simulink model "demonstrator"  (Simulink 7.4)
settings: Solver=FixedStepDiscrete  StartTime=0.0  StopTime=10.0  FixedStep=0.001  RelTol=1e-3
libraries: BusImpl x3, AtomicLibrary x1, robot x1, robot2 x1
settings Model: Creator=andrey  LastModifiedBy=andrey
settings SolverCC: AutoInsertRateTranBlk=on
settings DebuggingCC: MultiTaskDSMMsg=warning  MultiTaskCondExecSysMsg=none
settings RTWCC: IncludeERTFirstTime=on

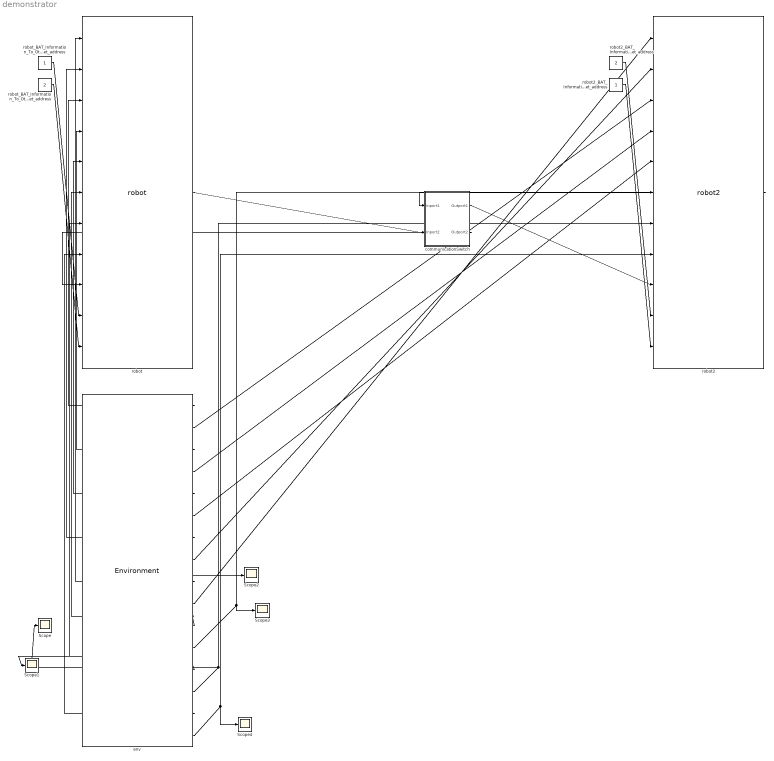
== system demonstrator ==
  Scope{,1..4} (5 alike) : Scope
      Scope settings: YMin=-1  YMax=1
      Scope1 settings: YMin=-1  YMax=1
      Scope2 settings: SaveName=ScopeData2
      Scope3 settings: YMin=-1  YMax=1  SaveName=ScopeData3
      Scope4 settings: YMin=-1  YMax=1  SaveName=ScopeData4
  communicationSwitch : Subsystem  Tag=id=_1766wKbHEeKVjd_905naCg  LoadFcn=MainBusGenerator
  env : AtomicLibrary/Environment  Tag=id=_2FmbMKbHEeKVjd_905naCg  SystemSampleTime=-1
  robot : robot/robot  Tag=id=_2BnTEKbHEeKVjd_905naCg  SystemSampleTime=-1
  robot2 : robot2/robot2  Tag=id=_2CgD4KbHEeKVjd_905naCg  SystemSampleTime=-1
  robot2_BAT_Information_To_OtherRobot_net_address : Constant  Tag=id=_3M3lQKbHEeKVjd_905naCg  Value=2  OutDataTypeMode=uint8  OutDataTypeStr=uint8
  robot2_BAT_Information_To_OtherRobot_send_receiver_net_address : Constant  Tag=id=_4yWVUabHEeKVjd_905naCg  OutDataTypeMode=uint8  OutDataTypeStr=uint8
  robot_BAT_Information_To_OtherRobot_net_address : Constant  Tag=id=_3Mo7wKbHEeKVjd_905naCg  OutDataTypeMode=uint8  OutDataTypeStr=uint8
  robot_BAT_Information_To_OtherRobot_send_receiver_net_address : Constant  Tag=id=_4yXjcabHEeKVjd_905naCg  Value=2  OutDataTypeMode=uint8  OutDataTypeStr=uint8
  wires:
  robot_BAT_Information_To_OtherRobot_net_address/1 -> robot/10
  robot2_BAT_Information_To_OtherRobot_net_address/1 -> robot2/10
  env/12 -> robot2/6, Scope3/1
  env/2 -> robot2/3
  env/3 -> robot/4
  env/9 -> robot/1
  env/10 -> robot2/1
  env/5 -> robot/5
  env/6 -> robot2/5
  env/11 -> robot/6, Scope2/1
  env/14 -> robot2/7, Scope/1
  env/8 -> robot2/2
  env/13 -> robot/7, Scope1/1
  env/1 -> robot/3
  env/7 -> robot/2
  env/4 -> robot2/4
  env/16 -> robot2/8, Scope4/1
  env/15 -> robot/8
  robot2/1 -> communicationSwitch/1(Inport1)
  robot/1 -> communicationSwitch/2(Inport2)
  communicationSwitch/2(Outport2) -> robot/9
  communicationSwitch/1(Outport1) -> robot2/9
  robot2_BAT_Information_To_OtherRobot_send_receiver_net_address/1 -> robot2/11
  robot_BAT_Information_To_OtherRobot_send_receiver_net_address/1 -> robot/11

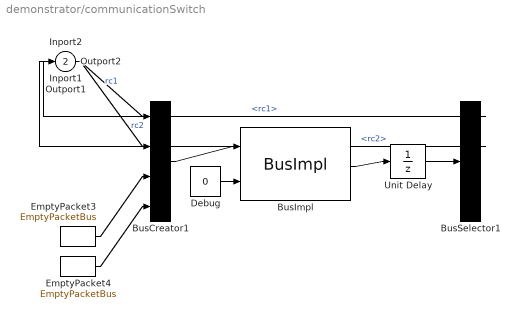
== system demonstrator/communicationSwitch ==
  Inport1 : Inport  Tag=id=_4yYKgKbHEeKVjd_905naCg  UseBusObject=on  OutDataType=fixdt(1, 16)  OutScaling=2^0
      settings: BusObject=PacketBus
  Inport2 : Inport  Tag=id=_4yYxkKbHEeKVjd_905naCg  Port=2  UseBusObject=on  OutDataType=fixdt(1, 16)  OutScaling=2^0
      settings: BusObject=PacketBus
  BusCreator1 : BusCreator  UseBusObject=on
      settings: BusObject=MainBus
  BusImpl : BusImpl/BusImpl  SystemSampleTime=-1
  BusSelector1 : BusSelector  OutputSignals=rc1,rc2,rc3,rc4
  Debug : Constant  Value=0  OutDataType=fixdt(1, 16)  OutScaling=2^0
  EmptyPacket3 : BusImpl/EmptyPacketBus  SystemSampleTime=-1
  EmptyPacket4 : BusImpl/EmptyPacketBus  SystemSampleTime=-1
  Unit Delay : UnitDelay  SampleTime=-1
  Outport1 : Outport  Tag=id=_4yYKgabHEeKVjd_905naCg  UseBusObject=on  OutDataType=fixdt(1, 16)  OutScaling=2^0
      settings: BusObject=PacketBus
  Outport2 : Outport  Tag=id=_4yYxkabHEeKVjd_905naCg  Port=2  UseBusObject=on  OutDataType=fixdt(1, 16)  OutScaling=2^0
      settings: BusObject=PacketBus
  wires:
  BusImpl/1 -> Unit Delay/1
  BusCreator1/1 -> BusImpl/1
  Unit Delay/1 -> BusSelector1/1
  Inport1/1 -> BusCreator1/1  "rc1"
  Inport2/1 -> BusCreator1/2  "rc2"
  BusSelector1/1 -> Outport1/1  "<rc1>"
  BusSelector1/2 -> Outport2/1  "<rc2>"
  Debug/1 -> BusImpl/2
  EmptyPacket3/1 -> BusCreator1/3
  EmptyPacket4/1 -> BusCreator1/4
